simulink model "ufunct"  (R2020a)
settings: Solver=VariableStepAuto  StartTime=0.0  StopTime=10.0  RelTol=1e-3
InitFcn:
  | I1 = 0.113;
  | L0 = 0.215;
  | tork = 1;
  | g = 9.81;
  | m1 = 5.38*10^(-2);
  | J1 =1.98*10^-4;
  | I0 = 1.75*10^-2;
undefined symbols (not defined in the file or in its folder): U
settings Model: Creator=muham  LastModifiedBy=muham

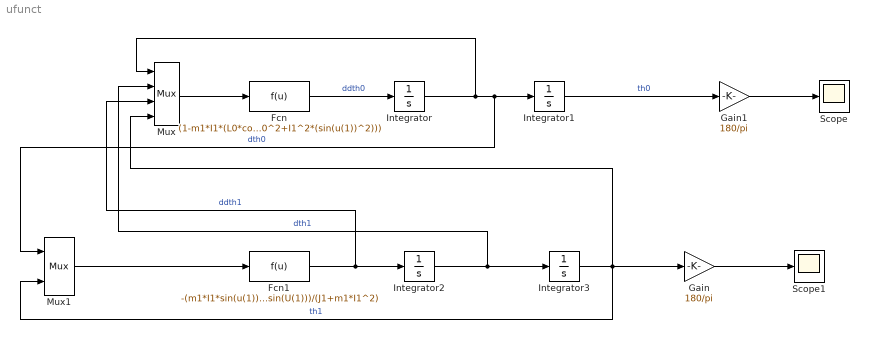
== system ufunct ==
  Fcn : Fcn  Expr=(1-m1*I1*(L0*cos(u(1)))*u(2)*sin(2*u(1))*u(3)*u(4)-L0*sin(u(1))*u(4)^2)/(I0+m1*(L0^2+I1^2*(sin(u(1))^2)))
  Fcn1 : Fcn  Expr=-(m1*I1*sin(u(1))*cos(u(1))*u(2)^2*g*sin(U(1)))/(J1+m1*I1^2)
  Gain : Gain  Gain=180/pi
  Gain1 : Gain  Gain=180/pi
  Integrator{,1..3} (4 alike) : Integrator
  Mux : Mux
  Mux1 : Mux  Inputs=2
  Scope : Scope
  Scope1 : Scope
  wires:
  Fcn/1 -> Integrator/1  "ddth0"
  Integrator/1 -> Mux/1, Mux1/1, Integrator1/1  "dth0"
  Integrator2/1 -> Mux/2, Integrator3/1  "dth1"
  Fcn1/1 -> Mux/3, Integrator2/1  "ddth1"
  Mux/1 -> Fcn/1
  Integrator3/1 -> Mux1/2, Gain/1, Mux/4  "th1"
  Mux1/1 -> Fcn1/1
  Integrator1/1 -> Gain1/1  "th0"
  Gain1/1 -> Scope/1
  Gain/1 -> Scope1/1
